simulink model "myproject_task"  (Simulink 3.00)
undefined symbols (not defined in the file): Double, F64
libraries: logiclib x20, execlib x10, langlib x3, matrixlib x3, arclib x3, mathlib x1
settings Model: MaskType=REX sequence  MaskIconFrame=on  MaskIconOpaque=on  MaskIconRotate=none  MaskIconUnits=autoscale

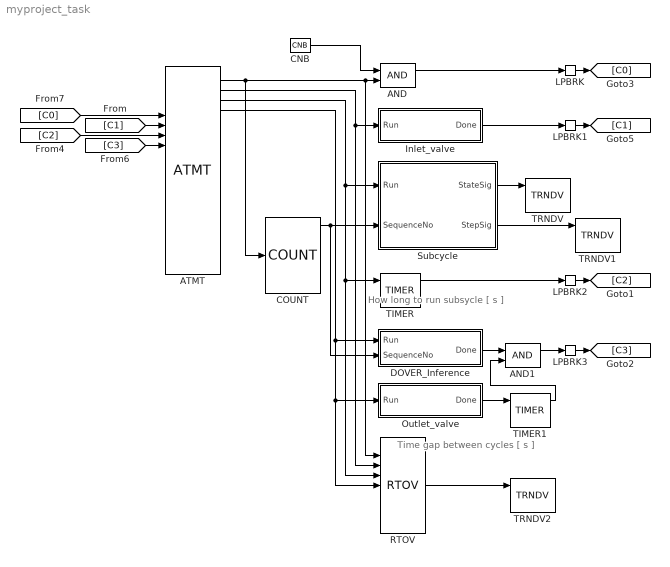
== system myproject_task ==
  note: How long to run subsycle [ s ]
  note: Time gap between cycles [ s ]
  AND : logiclib/AND
  AND1 : logiclib/AND
  ATMT : logiclib/ATMT  morestps=off  STT=[0 0 1; 1 1 2; 2 2 3; 3 3 0]  touts=[1 2 3 4 5 6 7 8 9 10 11 12 13 14 15 16]
  CNB : mathlib/CNB  YCN=on
  COUNT : logiclib/COUNT
  DOVER_Inference : Subsystem
      mask Type: REX sequence
  Inlet_valve : Subsystem
      mask Type: REX sequence
  LPBRK{,1..3} (4 alike) : execlib/LPBRK  RB=off
  Outlet_valve : Subsystem
      mask Type: REX sequence
  RTOV : matrixlib/RTOV  nmax=8  offset=0  n=8  etype=8: Double (F64)
  Subcycle : Subsystem
      mask Type: REX sequence
  TIMER : logiclib/TIMER  mode=2: Delayed ON  pt=30
  TIMER1 : logiclib/TIMER  mode=2: Delayed ON  pt=1
  TRNDV : arclib/TRNDV  n=8  l=1000  btype=8: Double (F64)  pfac=1  afac=1  arc=0  id=1  title=Trend Title  timesrc=1: CORETIMER
  TRNDV1 : arclib/TRNDV  n=8  l=1000  btype=8: Double (F64)  pfac=1  afac=1  arc=0  id=1  title=Trend Title  timesrc=1: CORETIMER
  TRNDV2 : arclib/TRNDV  n=8  l=1000  btype=8: Double (F64)  pfac=1  afac=1  arc=0  id=1  title=Trend Title  timesrc=1: CORETIMER
  wires:
  AND/1 -> LPBRK/1
  AND1/1 -> LPBRK3/1
  ATMT/1 -> AND/2, RTOV/2, COUNT/4
  ATMT/2 -> Inlet_valve/1(Run), RTOV/3
  ATMT/3 -> Subcycle/1(Run), RTOV/4, TIMER/1
  ATMT/4 -> Outlet_valve/1(Run), RTOV/5, DOVER_Inference/1(Run)
  CNB/1 -> AND/1
  COUNT/1 -> DOVER_Inference/2(SequenceNo), Subcycle/2(SequenceNo)
  DOVER_Inference/1(Done) -> AND1/1
  [C1] -> ATMT/6
  [C2] -> ATMT/7
  [C3] -> ATMT/8
  [C0] -> ATMT/5
  Inlet_valve/1(Done) -> LPBRK1/1
  LPBRK/1 -> [C0]
  LPBRK1/1 -> [C1]
  LPBRK2/1 -> [C2]
  LPBRK3/1 -> [C3]
  Outlet_valve/1(Done) -> TIMER1/1
  RTOV/1 -> TRNDV2/1
  Subcycle/1(StateSig) -> TRNDV/1
  Subcycle/2(StepSig) -> TRNDV1/1
  TIMER/1 -> LPBRK2/1
  TIMER1/1 -> AND1/2

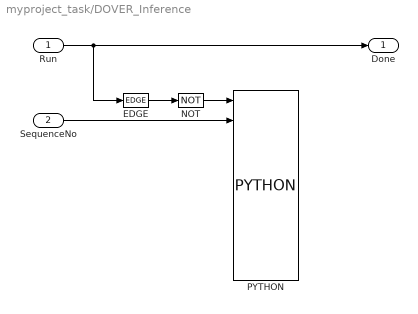
== system myproject_task/DOVER_Inference ==
  Run : Inport  Port=1  OutDataTypeStr=Inherit: auto
  SequenceNo : Inport  Port=2  OutDataTypeStr=Inherit: auto
  EDGE : logiclib/EDGE  iedge=1: Rising edge
  NOT : logiclib/NOT
  PYTHON : langlib/PYTHON  srcname=inference_dover_onnx.py  embedded=on  p0=/mnt/external_hdd/DoverRexTest  p1=dover_mobile  p2=onnxruntime  p3=/mnt/external_hdd/ATMTRexTest/sequences  p4=16
  Done : Outport  Port=1  OutDataTypeStr=Inherit: auto
  wires:
  EDGE/1 -> NOT/1
  NOT/1 -> PYTHON/1
  Run/1 -> Done/1, EDGE/1
  SequenceNo/1 -> PYTHON/3

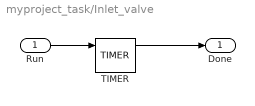
== system myproject_task/Inlet_valve ==
  Run : Inport  Port=1  OutDataTypeStr=Inherit: auto
  TIMER : logiclib/TIMER  mode=2: Delayed ON  pt=10
  Done : Outport  Port=1  OutDataTypeStr=Inherit: auto
  wires:
  Run/1 -> TIMER/1
  TIMER/1 -> Done/1

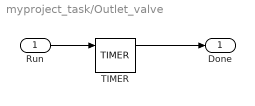
== system myproject_task/Outlet_valve ==
  Run : Inport  Port=1  OutDataTypeStr=Inherit: auto
  TIMER : logiclib/TIMER  mode=2: Delayed ON  pt=10
  Done : Outport  Port=1  OutDataTypeStr=Inherit: auto
  wires:
  Run/1 -> TIMER/1
  TIMER/1 -> Done/1

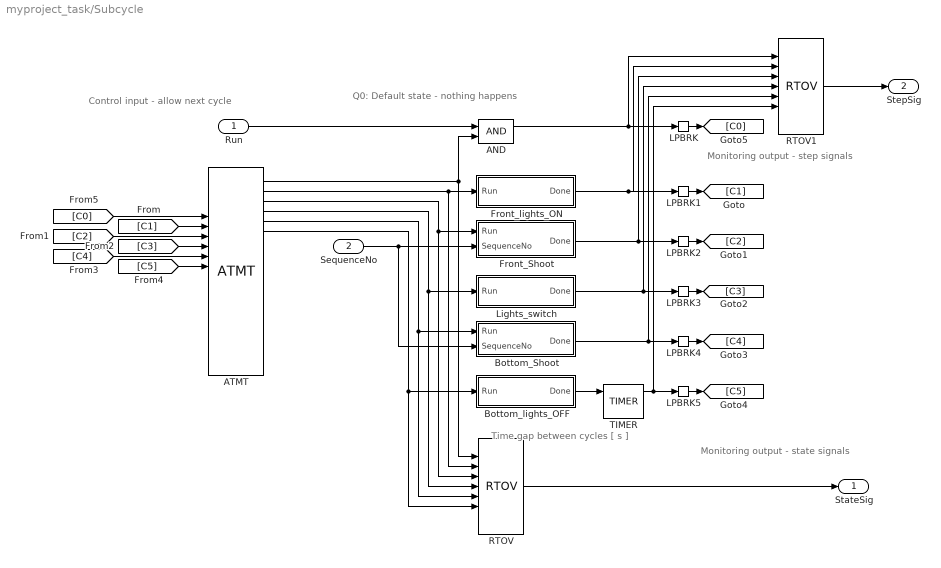
== system myproject_task/Subcycle ==
  note: Q0: Default state - nothing happens
  note: Control input - allow next cycle
  note: Monitoring output - step signals
  note: Monitoring output - state signals
  note: Time gap between cycles [ s ]
  Run : Inport  Port=1  OutDataTypeStr=Inherit: auto
  SequenceNo : Inport  Port=2  OutDataTypeStr=Inherit: auto
  AND : logiclib/AND
  ATMT : logiclib/ATMT  morestps=off  STT=[0 0 1; 1 1 2; 2 2 3; 3 3 4; 4 4 5; 5 5 0]  touts=[ 0 0 0 0 0 0 0 0 0 0 0 0 0 0 0 0]
  Bottom_Shoot : Subsystem
      mask Type: REX sequence
  Bottom_lights_OFF : Subsystem
      mask Type: REX sequence
  Front_Shoot : Subsystem
      mask Type: REX sequence
  Front_lights_ON : Subsystem
      mask Type: REX sequence
  LPBRK{,1..5} (6 alike) : execlib/LPBRK  RB=off
  Lights_switch : Subsystem
      mask Type: REX sequence
  RTOV : matrixlib/RTOV  nmax=8  offset=0  n=8  etype=8: Double (F64)
  RTOV1 : matrixlib/RTOV  nmax=8  offset=0  n=8  etype=8: Double (F64)
  TIMER : logiclib/TIMER  mode=2: Delayed ON  pt=0
  StateSig : Outport  Port=1  OutDataTypeStr=Inherit: auto
  StepSig : Outport  Port=2  OutDataTypeStr=Inherit: auto
  wires:
  AND/1 -> LPBRK/1, RTOV1/2
  ATMT/1 -> AND/2, RTOV/2
  ATMT/2 -> Front_lights_ON/1(Run), RTOV/3
  ATMT/3 -> Front_Shoot/1(Run), RTOV/4
  ATMT/4 -> Lights_switch/1(Run), RTOV/5
  ATMT/5 -> Bottom_Shoot/1(Run), RTOV/6
  ATMT/6 -> Bottom_lights_OFF/1(Run), RTOV/7
  Bottom_Shoot/1(Done) -> LPBRK4/1, RTOV1/6
  Bottom_lights_OFF/1(Done) -> TIMER/1
  [C1] -> ATMT/6
  [C2] -> ATMT/7
  [C3] -> ATMT/8
  [C4] -> ATMT/9
  [C5] -> ATMT/10
  [C0] -> ATMT/5
  Front_Shoot/1(Done) -> LPBRK2/1, RTOV1/4
  Front_lights_ON/1(Done) -> LPBRK1/1, RTOV1/3
  LPBRK/1 -> [C0]
  LPBRK1/1 -> [C1]
  LPBRK2/1 -> [C2]
  LPBRK3/1 -> [C3]
  LPBRK4/1 -> [C4]
  LPBRK5/1 -> [C5]
  Lights_switch/1(Done) -> LPBRK3/1, RTOV1/5
  RTOV/1 -> StateSig/1
  RTOV1/1 -> StepSig/1
  Run/1 -> AND/1
  SequenceNo/1 -> Bottom_Shoot/2(SequenceNo), Front_Shoot/2(SequenceNo)
  TIMER/1 -> LPBRK5/1, RTOV1/7

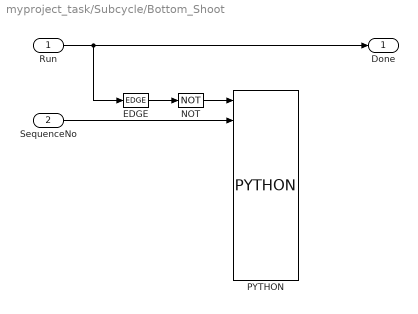
== system myproject_task/Subcycle/Bottom_Shoot ==
  Run : Inport  Port=1  OutDataTypeStr=Inherit: auto
  SequenceNo : Inport  Port=2  OutDataTypeStr=Inherit: auto
  EDGE : logiclib/EDGE  iedge=1: Rising edge
  NOT : logiclib/NOT
  PYTHON : langlib/PYTHON  srcname=shoot.py  embedded=on  p0=/mnt/external_hdd/ATMTRexTest/sequences  p1=bottom  p2=1  p3=1000  p4=10
  Done : Outport  Port=1  OutDataTypeStr=Inherit: auto
  wires:
  EDGE/1 -> NOT/1
  NOT/1 -> PYTHON/1
  Run/1 -> Done/1, EDGE/1
  SequenceNo/1 -> PYTHON/3

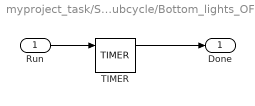
== system myproject_task/Subcycle/Bottom_lights_OFF ==
  Run : Inport  Port=1  OutDataTypeStr=Inherit: auto
  TIMER : logiclib/TIMER  mode=2: Delayed ON  pt=1
  Done : Outport  Port=1  OutDataTypeStr=Inherit: auto
  wires:
  Run/1 -> TIMER/1
  TIMER/1 -> Done/1

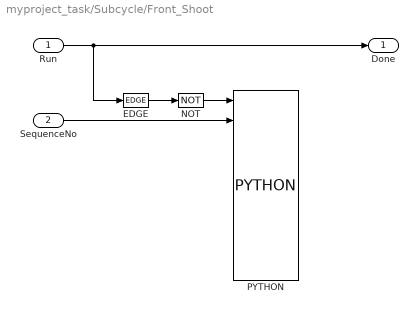
== system myproject_task/Subcycle/Front_Shoot ==
  Run : Inport  Port=1  OutDataTypeStr=Inherit: auto
  SequenceNo : Inport  Port=2  OutDataTypeStr=Inherit: auto
  EDGE : logiclib/EDGE  iedge=1: Rising edge
  NOT : logiclib/NOT
  PYTHON : langlib/PYTHON  srcname=shoot.py  embedded=on  p0=/mnt/external_hdd/ATMTRexTest/sequences  p1=front  p2=1  p3=1000  p4=10
  Done : Outport  Port=1  OutDataTypeStr=Inherit: auto
  wires:
  EDGE/1 -> NOT/1
  NOT/1 -> PYTHON/1
  Run/1 -> Done/1, EDGE/1
  SequenceNo/1 -> PYTHON/3

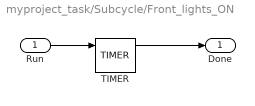
== system myproject_task/Subcycle/Front_lights_ON ==
  Run : Inport  Port=1  OutDataTypeStr=Inherit: auto
  TIMER : logiclib/TIMER  mode=2: Delayed ON  pt=1
  Done : Outport  Port=1  OutDataTypeStr=Inherit: auto
  wires:
  Run/1 -> TIMER/1
  TIMER/1 -> Done/1

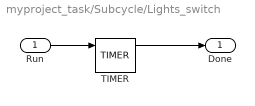
== system myproject_task/Subcycle/Lights_switch ==
  Run : Inport  Port=1  OutDataTypeStr=Inherit: auto
  TIMER : logiclib/TIMER  mode=2: Delayed ON  pt=1
  Done : Outport  Port=1  OutDataTypeStr=Inherit: auto
  wires:
  Run/1 -> TIMER/1
  TIMER/1 -> Done/1
